simulink subsystem "accSensor2CM"  (R2021a)
settings: Solver=VariableStepAuto  StartTime=0.0  StopTime=10.0  RelTol=1e-3
undefined symbols (not defined in the file): config
libraries: vrlib x3, attitude_library x3
settings Model: Creator=Laura  LastModifiedBy=Laura

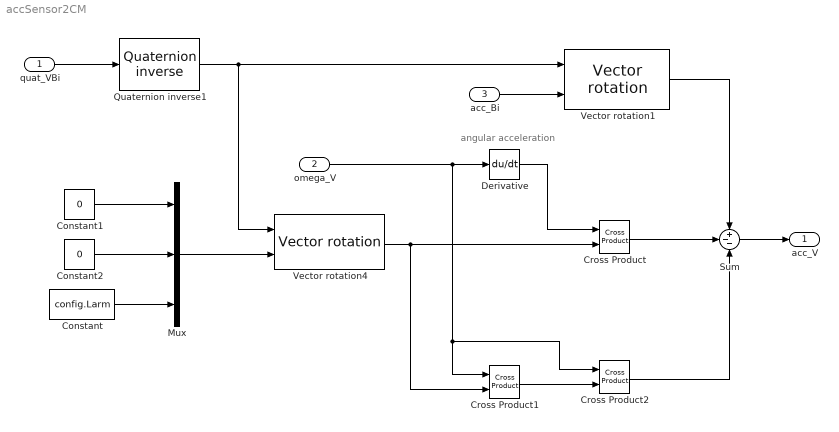
== system accSensor2CM ==
  note: angular acceleration
  quat_VBi : Inport
  omega_V : Inport  Port=2
  acc_Bi : Inport  Port=3
  Constant : Constant  Value=config.Larm
  Constant1 : Constant  Value=0
  Constant2 : Constant  Value=0
  Cross Product : vrlib/Utilities/Cross Product
  Cross Product1 : vrlib/Utilities/Cross Product
  Cross Product2 : vrlib/Utilities/Cross Product
  Derivative : Derivative
  Mux : Mux  Inputs=3
  Quaternion inverse1 : attitude_library/Quaternion inverse  SystemSampleTime=-1  VariantActivationTime=update diagram  Latency=0  AutoFrameSizeCalculation=off
      settings: SourceProductName=Attitude library
  Sum : Sum  Inputs=+--
  Vector rotation1 : attitude_library/Vector rotation  SystemSampleTime=-1  VariantActivationTime=update diagram  Latency=0  AutoFrameSizeCalculation=off
      settings: SourceProductName=Attitude library
  Vector rotation4 : attitude_library/Vector rotation  SystemSampleTime=-1  VariantActivationTime=update diagram  Latency=0  AutoFrameSizeCalculation=off
      settings: SourceProductName=Attitude library
  acc_V : Outport
  wires:
  Derivative/1 -> Cross Product/1
  Vector rotation1/1 -> Sum/1
  Constant/1 -> Mux/3
  omega_V/1 -> Cross Product1/1, Cross Product2/1, Derivative/1
  Cross Product/1 -> Sum/2
  acc_Bi/1 -> Vector rotation1/2
  Constant1/1 -> Mux/1
  Constant2/1 -> Mux/2
  Cross Product2/1 -> Sum/3
  Mux/1 -> Vector rotation4/2
  Cross Product1/1 -> Cross Product2/2
  Vector rotation4/1 -> Cross Product1/2, Cross Product/2
  Sum/1 -> acc_V/1
  Quaternion inverse1/1 -> Vector rotation4/1, Vector rotation1/1
  quat_VBi/1 -> Quaternion inverse1/1
